simulink model "Q2_W2"  (R2020b)
settings: Solver=VariableStepAuto  StartTime=0.0  StopTime=100  RelTol=1e-3
settings Model: Creator=hp  LastModifiedBy=hp

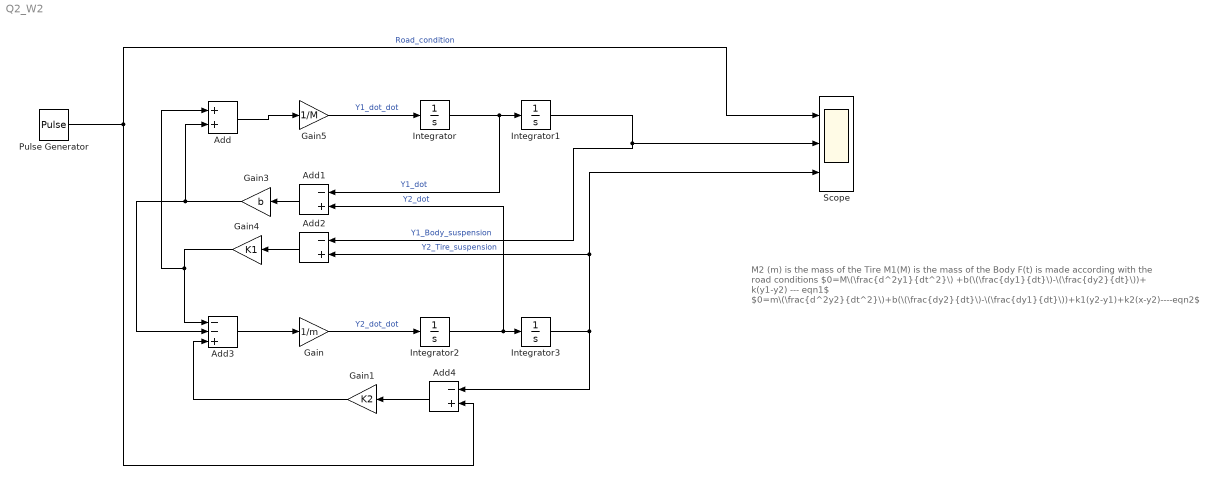
== system Q2_W2 ==
  note: M2 (m) is the mass of the Tire
      | M1(M) is the mass of the Body
      | F(t) is made according with the road conditions
      | $0=M\(\frac{d^2y1}{dt^2}\) +b(\(\frac{dy1}{dt}\)-\(\frac{dy2}{dt}\))+ k(y1-y2) --- eqn1$
      | $0=m\(\frac{d^2y2}{dt^2}\)+b(\(\frac{dy2}{dt}\)-\(\frac{dy1}{dt}\))+k1(y2-y1)+k2(x-y2)----eqn2$
  Add : Sum
  Add1 : Sum  Inputs=-+
  Add2 : Sum  Inputs=-+
  Add3 : Sum  Inputs=--+
  Add4 : Sum  Inputs=-+
  Gain : Gain  Gain=1/m  mask{m=20}
  Gain1 : Gain  Gain=K2  mask{K2=1000}
  Gain3 : Gain  Gain=b  mask{b=500}
  Gain4 : Gain  Gain=K1  mask{K1=500}
  Gain5 : Gain  Gain=1/M  mask{M=500}
  Integrator{,1..3} (4 alike) : Integrator
  Pulse Generator : DiscretePulseGenerator  PulseType=Time based  Period=40  PulseWidth=20
  Scope : Scope  NumInputPorts=3
  wires:
  Add/1 -> Gain5/1
  Gain5/1 -> Integrator/1  "Y1_dot_dot"
  Integrator/1 -> Add1/1, Integrator1/1  "Y1_dot"
  Integrator1/1 -> Add2/1, Scope/2  "Y1_Body_suspension"
  Add3/1 -> Gain/1
  Gain/1 -> Integrator2/1  "Y2_dot_dot"
  Integrator2/1 -> Add1/2, Integrator3/1  "Y2_dot"
  Integrator3/1 -> Add4/1, Scope/3, Add2/2  "Y2_Tire_suspension"
  Add1/1 -> Gain3/1
  Add2/1 -> Gain4/1
  Gain1/1 -> Add3/3
  Gain3/1 -> Add/2, Add3/2
  Gain4/1 -> Add/1, Add3/1
  Add4/1 -> Gain1/1
  Pulse Generator/1 -> Scope/1, Add4/2  "Road_condition"
